simulink model "Communication"  (R2020b)
settings: Solver=VariableStepAuto  StartTime=0.0  StopTime=10.0  RelTol=1e-3
libraries: opclib x3
settings Model: Creator=Asus  LastModifiedBy=Asus

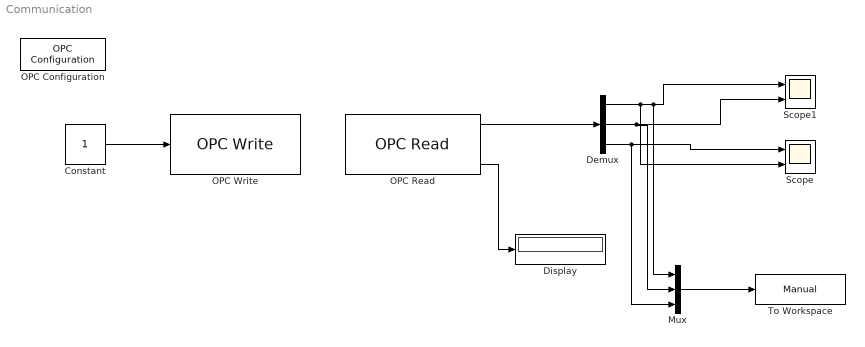
== system Communication ==
  Constant : Constant  VectorParams1D=off  SampleTime=-1
  Demux : Demux  Outputs=3
  Display : Display
  Mux : Mux  Inputs=3
  OPC Configuration : opclib/OPC Configuration  errMissingItems=Error  errReadWrite=Warn  errShutdown=Error  errRTViolation=Warn  rtEnable=on  speedup=1  showLatency=off  beingUsed=on
      settings: SourceProductBaseCode=OT
  OPC Read : opclib/OPC Read  readMode=Synchronous (cache)  dataType=double  updateRate=0.5  showQual=on  showTS=on  tsMode=Seconds since start
      settings: SourceProductBaseCode=OT
  OPC Write : opclib/OPC Write  writeMode=Synchronous  updateRate=0
      settings: SourceProductBaseCode=OT
  Scope : Scope  NumInputPorts=2
  Scope1 : Scope  NumInputPorts=2
  To Workspace : ToWorkspace  VariableName=Manual  SaveFormat=Timeseries  SampleTime=-1
  wires:
  OPC Read/1 -> Demux/1
  Demux/2 -> Mux/2, Scope1/2
  Demux/1 -> Scope/2, Mux/1, Scope1/1
  Demux/3 -> Mux/3, Scope/1
  Constant/1 -> OPC Write/1
  Mux/1 -> To Workspace/1
  OPC Read/3 -> Display/1
